simulink model "Nelinearni_test"  (R2023b)
settings: Solver=VariableStepAuto  StartTime=0.0  StopTime=stepp.sim_time  RelTol=1e-3
undefined symbols (not defined in the file or in its folder): boost, Ci, m0_ccm, Ramp, sim_op, stepp
libraries: spsSeriesRLCBranchLib x6, spsCurrentMeasurementLib x4, spsVoltageMeasurementLib x2, dspstat3 x2, spsControlledVoltageSourceLib x1, spsDiodeLib x1, spsIdealSwitchLib x1, spsBistableLib x1, simulink x1, sps_lib x1
settings Model: Creator=teo  LastModifiedBy=teo

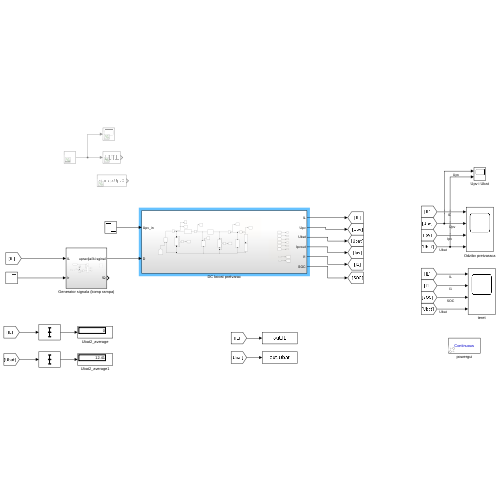
[thumbnail: Simulink's stored preview of the top-level diagram]
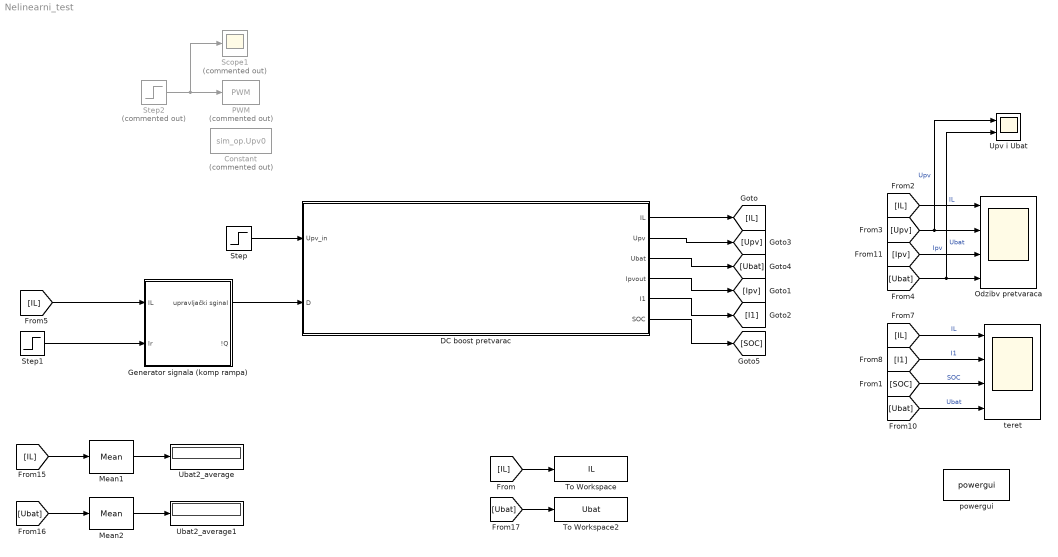
== system Nelinearni_test ==
  Constant : Constant  Commented=on  Value=sim_op.Upv0
  DC boost pretvarac : Subsystem
  Generator signala (komp rampa) : Subsystem
  Mean1 : dspstat3/Mean  run=off  InputProcessing=Columns as channels (frame based)  reset_popup=None  directionMode=Entire input  dimension=1  roiEnable=off  roiType=Rectangles  roiPortion=Entire ROI  roiOutput=Individual statistics for each ROI  roiFlag=off  roundingMode=Floor  overflowMode=off  outputDataTypeStr=Inherit: Same as accumulator  outputMin=[]  outputMax=[]  outputLastDataTypeStr=Inherit: Same as accumulator
  Mean2 : dspstat3/Mean  run=off  InputProcessing=Columns as channels (frame based)  reset_popup=None  directionMode=Entire input  dimension=1  roiEnable=off  roiType=Rectangles  roiPortion=Entire ROI  roiOutput=Individual statistics for each ROI  roiFlag=off  roundingMode=Floor  overflowMode=off  outputDataTypeStr=Inherit: Same as accumulator  outputMin=[]  outputMax=[]  outputLastDataTypeStr=Inherit: Same as accumulator
  Odzibv pretvaraca : Scope  NumInputPorts=4
  PWM : simulink/Discontinuities/PWM  Commented=on  DisableCoverage=on  Period=boost.T  InitialDelay=0  DisallowZeroDutyCycle=off  RunAtFixedTimeIntervals=off  SampleTime=0.1
  Scope1 : Scope  Commented=on
  Step : Step  Time=stepp.step_time  Before=stepp.upv1  After=stepp.upv2  SampleTime=0
  Step1 : Step  Time=stepp.step_time  Before=stepp.ir01  After=stepp.ir02  SampleTime=0
  Step2 : Step  Commented=on  Time=stepp.step_time  Before=stepp.d1  After=stepp.d2  SampleTime=0
  To Workspace : ToWorkspace  VariableName=IL  SaveFormat=Timeseries  SampleTime=1e-6
  To Workspace2 : ToWorkspace  VariableName=Ubat  SaveFormat=Timeseries  SampleTime=1e-6
  Ubat2_average : Display
  Ubat2_average1 : Display
  Upv i Ubat : Scope  NumInputPorts=2
  powergui : sps_lib/powergui  Priority=1  SimulationMode=Continuous  SampleTime=50e-6  frequency=60  Iterations=50  frequencyindice=0  Pbase=100e6  ErrMax=1e-4  UnitsV=kV  UnitsW=MW  buscounter=0  FunctionMessages=off  echomessages=off  EnableUseOfTLC=off  CurrentSourceSwitches=off  DisableSnubberDevices=off  DisableRonSwitches=off  DisableVfSwitches=off  DisplayEquations=off  AutomaticDiscreteSolvers=off  SolverType=Tustin/Backward Euler (TBE)  Interpol=off  ExternalGateDelay=off  methode=off  Ts=100  x0status=blocks  SPID=on  SwTol=0  HookPort=off  NonlinearTolerance=1e-4  nMaxIteration=100  ContinueOnMaxIteration=off  RestoreLinks=warning  ResistiveCurrentMeasurement=off  Frange=[0:2:500]  Ylog=off  Xlog=on  ShowGrid=off  save=off  variable=ZData  structure=0  ZoomFFT=off  StartTime=0.0  cycles=1  DisplayStyle=1  fundamental=60  FreqAxis=off  MaxFrequency=1000  frequencyindicesteady=1  RmsSteady=1  display=off
  teret : Scope  NumInputPorts=4
  wires:
  Mean1/1 -> Ubat2_average/1
  [Ubat] -> To Workspace2/1
  [I1] -> teret/2  "I1"
  [Ubat] -> Mean2/1
  [Ubat] -> Upv i Ubat/2, Odzibv pretvaraca/4  "Ubat"
  [Upv] -> Upv i Ubat/1, Odzibv pretvaraca/2  "Upv"
  [IL] -> Mean1/1
  [Ipv] -> Odzibv pretvaraca/3  "Ipv"
  [IL] -> teret/1  "IL"
  [IL] -> To Workspace/1
  Mean2/1 -> Ubat2_average1/1
  [IL] -> Odzibv pretvaraca/1  "IL"
  [Ubat] -> teret/4  "Ubat"
  DC boost pretvarac/1(IL) -> [IL]
  DC boost pretvarac/2(Upv) -> [Upv]
  DC boost pretvarac/3(Ubat) -> [Ubat]
  DC boost pretvarac/4(Ipvout) -> [Ipv]
  DC boost pretvarac/5(I1) -> [I1]
  DC boost pretvarac/6(SOC) -> [SOC]
  [SOC] -> teret/3  "SOC"
  Step1/1 -> Generator signala (komp rampa)/2(Ir)
  [IL] -> Generator signala (komp rampa)/1(IL)
  Step2/1 -> Scope1/1, PWM/1
  Generator signala (komp rampa)/1(upravljački sginal) -> DC boost pretvarac/2(D)
  Step/1 -> DC boost pretvarac/1(Upv_in)

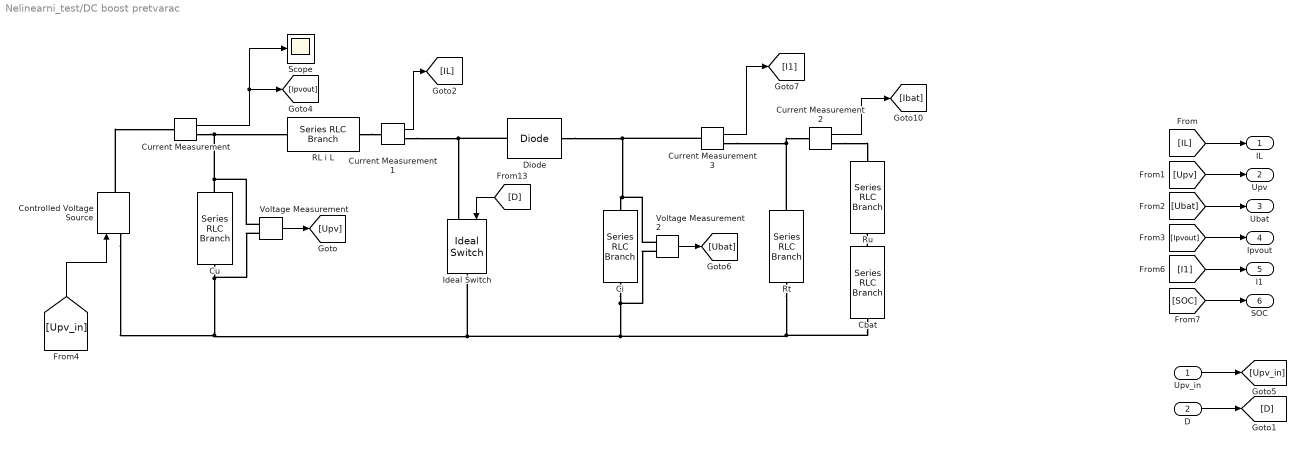
== system Nelinearni_test/DC boost pretvarac ==
  Upv_in : Inport
  D : Inport  Port=2
  Cbat : spsSeriesRLCBranchLib/Series RLC Branch  LConnTagsString=__new0  RConnTagsString=__new0  BranchType=C  Resistance=0.001  Inductance=1e-3  SetiL0=off  InitialCurrent=0  Capacitance=1*10^4  Setx0=on  InitialVoltage=sim_op.Ubat0 - 0.32  Measurements=None
  Ci : spsSeriesRLCBranchLib/Series RLC Branch  LConnTagsString=__new0  RConnTagsString=__new0  BranchType=C  Resistance=0.001  Inductance=1e-3  SetiL0=off  InitialCurrent=0  Capacitance=boost.Ci  Setx0=on  InitialVoltage=sim_op.Ubat0 - 0.32  Measurements=None
  Controlled Voltage Source : spsControlledVoltageSourceLib/Controlled Voltage Source  Initialize=on  Source_Type=AC  Amplitude=0  Phase=0  Frequency=0  Measurements=None
  Cu : spsSeriesRLCBranchLib/Series RLC Branch  LConnTagsString=__new0  RConnTagsString=__new0  BranchType=RC  Resistance=0.001  Inductance=1e-3  SetiL0=off  InitialCurrent=0  Capacitance=boost.Cu  Setx0=on  InitialVoltage=sim_op.Upv0  Measurements=None
  Current Measurement{,1..3} (4 alike) : spsCurrentMeasurementLib/Current Measurement  PhasorSimulation=off  OutputType=Complex  PSBequivalent=0
  Diode : spsDiodeLib/Diode  Ron=0  Lon=0  Vf=0  IC=0  UseSnubber=0  Rs=0  Cs=0  Measurements=off
  Ideal Switch : spsIdealSwitchLib/Ideal Switch  Ron=0  Lon=0  IC=0  Rs=0  Cs=0  Measurements=off
  RL i L : spsSeriesRLCBranchLib/Series RLC Branch  LConnTagsString=__new0  RConnTagsString=__new0  BranchType=RL  Resistance=boost.RL  Inductance=boost.L  SetiL0=off  InitialCurrent=stepp.ir01  Capacitance=1e-6  Setx0=off  InitialVoltage=0  Measurements=None
  Rt : spsSeriesRLCBranchLib/Series RLC Branch  LConnTagsString=__new0  RConnTagsString=__new0  BranchType=R  Resistance=boost.Rt  Inductance=1e-3  SetiL0=off  InitialCurrent=0  Capacitance=Ci  Setx0=off  InitialVoltage=0  Measurements=None
  Ru : spsSeriesRLCBranchLib/Series RLC Branch  LConnTagsString=__new0  RConnTagsString=__new0  BranchType=R  Resistance=boost.Ru  Inductance=1e-3  SetiL0=off  InitialCurrent=0  Capacitance=Ci  Setx0=off  InitialVoltage=0  Measurements=None
  Scope : Scope
  Voltage Measurement : spsVoltageMeasurementLib/Voltage Measurement  PhasorSimulation=off  OutputType=Complex  PSBequivalent=0
  Voltage Measurement2 : spsVoltageMeasurementLib/Voltage Measurement  PhasorSimulation=off  OutputType=Complex  PSBequivalent=0
  IL : Outport
  Upv : Outport  Port=2
  Ubat : Outport  Port=3
  Ipvout : Outport  Port=4
  I1 : Outport  Port=5
  SOC : Outport  Port=6
  wires:
  Current Measurement1/1 -> [IL]
  Voltage Measurement/1 -> [Upv]
  [D] -> Ideal Switch/1
  D/1 -> [D]
  Upv_in/1 -> [Upv_in]
  [IL] -> IL/1
  [Upv] -> Upv/1
  [Ubat] -> Ubat/1
  Current Measurement/1 -> Scope/1, [Ipvout]
  [Ipvout] -> Ipvout/1
  [I1] -> I1/1
  Voltage Measurement2/1 -> [Ubat]
  Current Measurement2/1 -> [Ibat]
  Current Measurement3/1 -> [I1]
  [SOC] -> SOC/1
  [Upv_in] -> Controlled Voltage Source/1
  connections:
  Current Measurement/RConn1 -- Voltage Measurement/LConn1 -- Cu/LConn1 -- RL i L/LConn1
  RL i L/RConn1 -- Current Measurement1/LConn1
  Diode/LConn1 -- Ideal Switch/LConn1 -- Current Measurement1/RConn1
  Ci/RConn1 -- Voltage Measurement2/LConn2 -- Cbat/RConn1 -- Rt/RConn1 -- Controlled Voltage Source/LConn1 -- Voltage Measurement/LConn2 -- Cu/RConn1 -- Ideal Switch/RConn1
  Voltage Measurement2/LConn1 -- Current Measurement3/LConn1 -- Diode/RConn1 -- Ci/LConn1
  Rt/LConn1 -- Current Measurement3/RConn1 -- Current Measurement2/LConn1
  Cbat/LConn1 -- Ru/RConn1
  Current Measurement2/RConn1 -- Ru/LConn1
  Controlled Voltage Source/RConn1 -- Current Measurement/LConn1

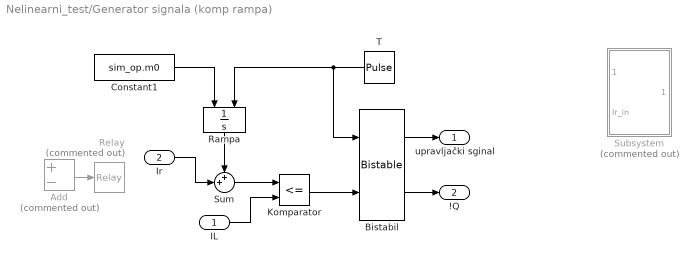
== system Nelinearni_test/Generator signala (komp rampa) ==
  IL : Inport
  Ir : Inport  Port=2
  Add : Sum  Commented=on  Inputs=+-
  Bistabil : spsBistableLib/Bistable  Qpriority=Set  ic=0  Ts=0
      settings: LibrarySourceBlock=sps_lib/Control/Bistable
  Constant1 : Constant  Value=sim_op.m0
  Komparator : RelationalOperator  Operator=<=  OutDataTypeStr=boolean  RndMeth=Simplest  InputSameDT=off
  Rampa : Integrator  ExternalReset=rising
  Relay : Relay  Commented=on  OnSwitchValue=0  OffSwitchValue=0
  Subsystem : Subsystem  Commented=on
  Sum : Sum  Inputs=++|
  T : DiscretePulseGenerator  PulseType=Time based  Period=boost.T
  upravljački sginal : Outport
  !Q : Outport  Port=2
  wires:
  Bistabil/2 -> !Q/1
  Bistabil/1 -> upravljački sginal/1
  Ir/1 -> Sum/2
  Rampa/1 -> Sum/1
  T/1 -> Bistabil/1, Rampa/2
  Constant1/1 -> Rampa/1
  Add/1 -> Relay/1
  Sum/1 -> Komparator/1
  IL/1 -> Komparator/2
  Komparator/1 -> Bistabil/2

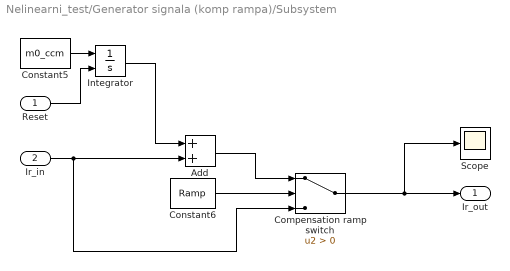
== system Nelinearni_test/Generator signala (komp rampa)/Subsystem ==
  Reset : Inport
  Ir_in : Inport  Port=2
  Add : Sum
  Compensation ramp switch : Switch  Criteria=u2 > Threshold  SaturateOnIntegerOverflow=off  InputSameDT=off
  Constant5 : Constant  Value=m0_ccm
  Constant6 : Constant  Value=Ramp
  Integrator : Integrator  ExternalReset=rising
  Scope : Scope
  Ir_out : Outport
  wires:
  Constant5/1 -> Integrator/1
  Integrator/1 -> Add/1
  Add/1 -> Compensation ramp switch/1
  Reset/1 -> Integrator/2
  Compensation ramp switch/1 -> Scope/1, Ir_out/1
  Constant6/1 -> Compensation ramp switch/2
  Ir_in/1 -> Compensation ramp switch/3, Add/2
